simulink model "sim_kajita_closed_loop"  (Simulink 8.5)
settings: Solver=ode45  StartTime=0.0  StopTime=10.0  RelTol=1e-3
values from neighbouring files (symbols this model uses):
  Br = [zeros(N-1,1); 1]    [PreviewControl.m]    (also in PreviewControl2.m)
  g = 9.81    [ComparingJacobians.m]    (also in avoidJointLimits.m = zeros(size(q)); changingmain.m)
  h = Plant.Ts    [PreviewControl.m]    (also in PreviewControl2.m)
  M = total_mass    [PreviewControl.m]    (also in PreviewControl2.m; calculate_inertia_matrix.m = zeros(3,length(m_hat)))
  Mr = [zeros(N-1,1), eye(N-1); zeros(1,N-1), 0;]    [PreviewControl.m]    (also in PreviewControl2.m)
  N = step_time*2/(h)    [PreviewControl.m]    (also in PreviewControl2.m = 320)
  NXRef0 = get_reference_x((0:N-1)'*h )    [PreviewControl.m]    (also in PreviewControl2.m = get_reference_x((1:N)'*h ))
  NYRef0 = get_reference_y((0:N-1)'*h )    [PreviewControl.m]    (also in PreviewControl2.m = get_reference_y((1:N)'*h ))
  z_c = interp1(lt,z_c,t)    [diff_eq.m]    (also in diff_eqx.m)
  zG = P_COG(3,1)    [ComparingJacobians.m]    (also in changingmain.m)
undefined symbols (not defined in the file or in its folder): Des_T_Cx, Des_T_Cy, Kx, Ky, X0, X0Dot, Y0, Y0Dot

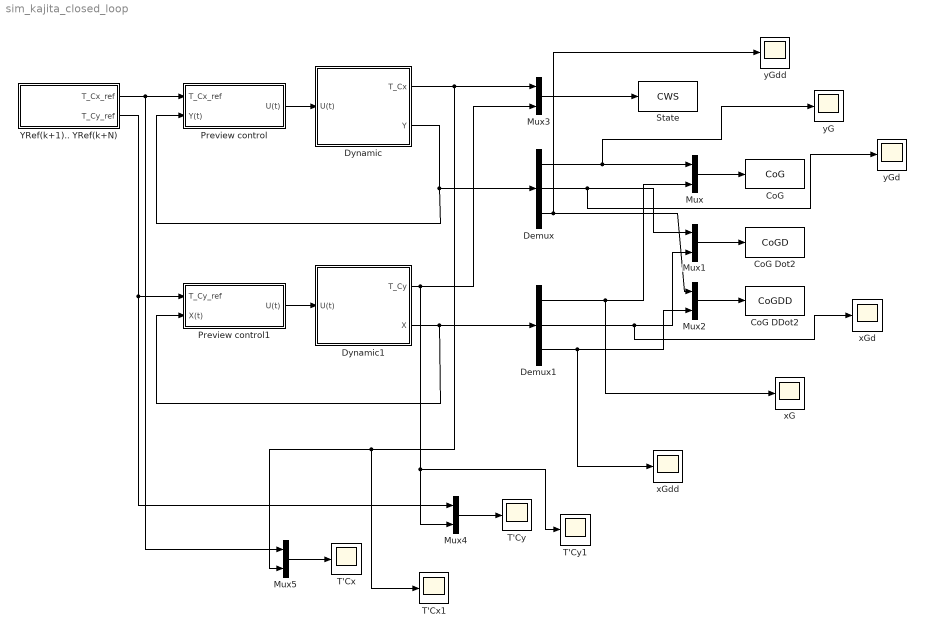
== system sim_kajita_closed_loop ==
  CoG : ToWorkspace  VariableName=CoG  SaveFormat=Structure With Time  SampleTime=-1
  CoG DDot2 : ToWorkspace  VariableName=CoGDD  SaveFormat=Structure With Time  SampleTime=-1
  CoG Dot2 : ToWorkspace  VariableName=CoGD  SaveFormat=Structure With Time  SampleTime=-1
  Demux : Demux  Outputs=3
  Demux1 : Demux  Outputs=3
  Dynamic : Subsystem
  Dynamic1 : Subsystem
  Mux{,1..5} (6 alike) : Mux  Inputs=2
  Preview control : Subsystem
  Preview control1 : Subsystem
  State : ToWorkspace  VariableName=CWS  SaveFormat=Structure With Time  SampleTime=-1
  T'Cx : Scope
  T'Cx1 : Scope
  T'Cy : Scope
  T'Cy1 : Scope
  YRef(k+1).. YRef(k+N) : Subsystem
  xG : Scope
  xGd : Scope
  xGdd : Scope
  yG : Scope
  yGd : Scope
  yGdd : Scope
  wires:
  Preview control/1(U(t)) -> Dynamic/1(U(t))
  Dynamic/2(Y) -> Preview control/2(Y(t)), Demux/1
  Demux/2 -> yGd/1, Mux1/1
  Demux/3 -> yGdd/1, Mux2/1
  Preview control1/1(U(t)) -> Dynamic1/1(U(t))
  Dynamic1/2(X) -> Preview control1/2(X(t)), Demux1/1
  Dynamic1/1(T_Cy) -> T'Cy1/1, Mux4/2, Mux3/2
  Demux1/2 -> xGd/1, Mux1/2
  YRef(k+1).. YRef(k+N)/2(T_Cy_ref) -> Mux4/1, Preview control1/1(T_Cy_ref)
  YRef(k+1).. YRef(k+N)/1(T_Cx_ref) -> Mux5/1, Preview control/1(T_Cx_ref)
  Demux/1 -> yG/1, Mux/1
  Demux1/1 -> xG/1, Mux/2
  Mux/1 -> CoG/1
  Mux2/1 -> CoG DDot2/1
  Demux1/3 -> xGdd/1, Mux2/2
  Mux1/1 -> CoG Dot2/1
  Mux3/1 -> State/1
  Dynamic/1(T_Cx) -> T'Cx1/1, Mux5/2, Mux3/1
  Mux4/1 -> T'Cy/1
  Mux5/1 -> T'Cx/1

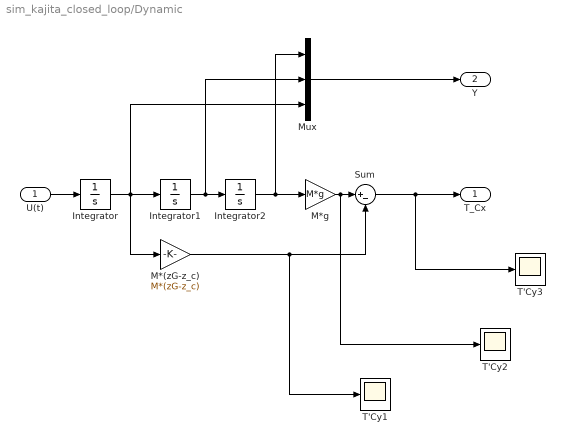
== system sim_kajita_closed_loop/Dynamic ==
  U(t) : Inport
  Integrator : Integrator
  Integrator1 : Integrator  InitialCondition=Y0Dot
  Integrator2 : Integrator  InitialCondition=Y0
  M*(zG-z_c) : Gain  Gain=M*(zG-z_c)
  M*g : Gain  Gain=M*g
  Mux : Mux  Inputs=3
  Sum : Sum  Inputs=|+-
  T'Cy1 : Scope
  T'Cy2 : Scope
  T'Cy3 : Scope
  T_Cx : Outport
  Y : Outport  Port=2
  wires:
  U(t)/1 -> Integrator/1
  Sum/1 -> T'Cy3/1, T_Cx/1
  Integrator/1 -> Integrator1/1, M*(zG-z_c)/1, Mux/3
  Integrator1/1 -> Integrator2/1, Mux/2
  Integrator2/1 -> M*g/1, Mux/1
  M*(zG-z_c)/1 -> T'Cy1/1, Sum/2
  Mux/1 -> Y/1
  M*g/1 -> T'Cy2/1, Sum/1

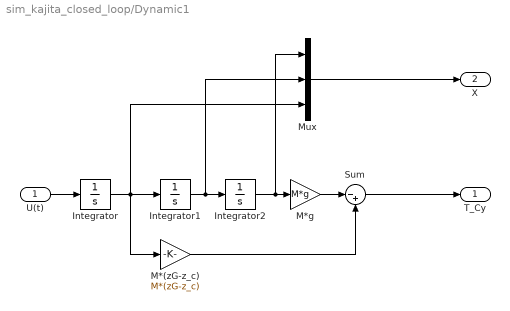
== system sim_kajita_closed_loop/Dynamic1 ==
  U(t) : Inport
  Integrator : Integrator
  Integrator1 : Integrator  InitialCondition=X0Dot
  Integrator2 : Integrator  InitialCondition=X0
  M*(zG-z_c) : Gain  Gain=M*(zG-z_c)
  M*g : Gain  Gain=M*g
  Mux : Mux  Inputs=3
  Sum : Sum  Inputs=|-+
  T_Cy : Outport
  X : Outport  Port=2
  wires:
  U(t)/1 -> Integrator/1
  Sum/1 -> T_Cy/1
  Integrator/1 -> Integrator1/1, M*(zG-z_c)/1, Mux/3
  Integrator1/1 -> Integrator2/1, Mux/2
  Integrator2/1 -> M*g/1, Mux/1
  M*(zG-z_c)/1 -> Sum/2
  Mux/1 -> X/1
  M*g/1 -> Sum/1

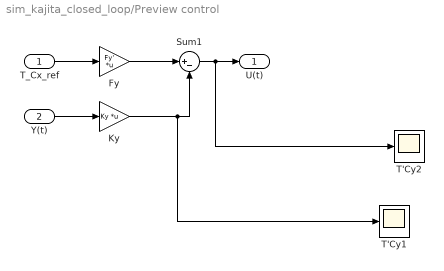
== system sim_kajita_closed_loop/Preview control ==
  T_Cx_ref : Inport
  Y(t) : Inport  Port=2
  Fy : Gain  Gain=Fy'  Multiplication=Matrix(K*u)
  Ky : Gain  Gain=Ky  Multiplication=Matrix(K*u)
  Sum1 : Sum  Inputs=|+-
  T'Cy1 : Scope
  T'Cy2 : Scope
  U(t) : Outport
  wires:
  Y(t)/1 -> Ky/1
  Ky/1 -> T'Cy1/1, Sum1/2
  Fy/1 -> Sum1/1
  T_Cx_ref/1 -> Fy/1
  Sum1/1 -> T'Cy2/1, U(t)/1

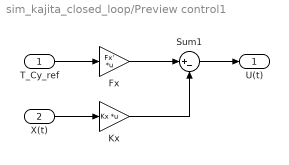
== system sim_kajita_closed_loop/Preview control1 ==
  T_Cy_ref : Inport
  X(t) : Inport  Port=2
  Fx : Gain  Gain=Fx'  Multiplication=Matrix(K*u)
  Kx : Gain  Gain=Kx  Multiplication=Matrix(K*u)
  Sum1 : Sum  Inputs=|+-
  U(t) : Outport
  wires:
  X(t)/1 -> Kx/1
  Kx/1 -> Sum1/2
  Fx/1 -> Sum1/1
  T_Cy_ref/1 -> Fx/1
  Sum1/1 -> U(t)/1

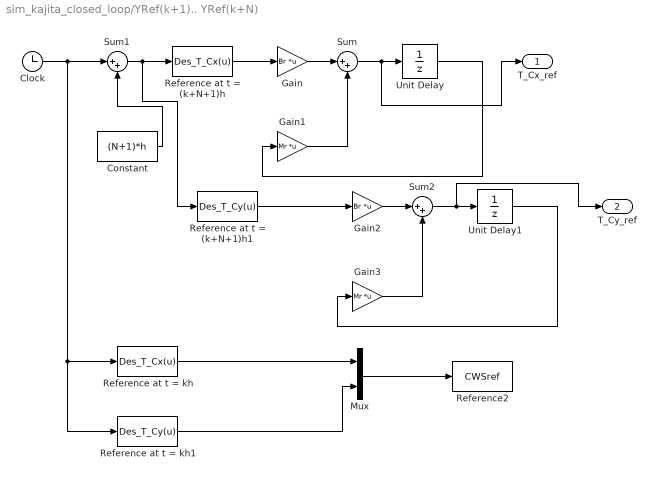
== system sim_kajita_closed_loop/YRef(k+1).. YRef(k+N) ==
  Clock : Clock
  Constant : Constant  Value=(N+1)*h
  Gain : Gain  Gain=Br  Multiplication=Matrix(K*u)
  Gain1 : Gain  Gain=Mr  Multiplication=Matrix(K*u)
  Gain2 : Gain  Gain=Br  Multiplication=Matrix(K*u)
  Gain3 : Gain  Gain=Mr  Multiplication=Matrix(K*u)
  Mux : Mux  Inputs=2
  Reference at t = (k+N+1)h : MATLABFcn  MATLABFcn=Des_T_Cx(u)
  Reference at t = (k+N+1)h1 : MATLABFcn  MATLABFcn=Des_T_Cy(u)
  Reference at t = kh : MATLABFcn  MATLABFcn=Des_T_Cx(u)  OutputDimensions=1
  Reference at t = kh1 : MATLABFcn  MATLABFcn=Des_T_Cy(u)  OutputDimensions=1
  Reference2 : ToWorkspace  VariableName=CWSref  SaveFormat=Structure With Time  SampleTime=-1
  Sum : Sum  Inputs=|++
  Sum1 : Sum  Inputs=|++
  Sum2 : Sum  Inputs=|++
  Unit Delay : UnitDelay  InitialCondition=NXRef0  SampleTime=h
  Unit Delay1 : UnitDelay  InitialCondition=NYRef0  SampleTime=h
  T_Cx_ref : Outport
  T_Cy_ref : Outport  Port=2
  wires:
  Gain/1 -> Sum/1
  Sum/1 -> T_Cx_ref/1, Unit Delay/1
  Gain1/1 -> Sum/2
  Unit Delay/1 -> Gain1/1
  Clock/1 -> Sum1/1, Reference at t = kh1/1, Reference at t = kh/1
  Constant/1 -> Sum1/2
  Sum1/1 -> Reference at t = (k+N+1)h/1, Reference at t = (k+N+1)h1/1
  Reference at t = (k+N+1)h/1 -> Gain/1
  Reference at t = kh/1 -> Mux/1
  Reference at t = kh1/1 -> Mux/2
  Gain2/1 -> Sum2/1
  Sum2/1 -> T_Cy_ref/1, Unit Delay1/1
  Gain3/1 -> Sum2/2
  Unit Delay1/1 -> Gain3/1
  Reference at t = (k+N+1)h1/1 -> Gain2/1
  Mux/1 -> Reference2/1
